simulink model "ECItoECEFtest"  (R2018a)
settings: Solver=FixedStepAuto  StartTime=0  StopTime=1*24*3600*365  FixedStep=10000  RelTol=1e-3
undefined symbols (not defined in the file or in its folder): Angle, Axis, IAU, init
libraries: robotcorelib x2, aerolibtransform2 x1, sharedtransform x1
settings Model: Creator=nathan  LastModifiedBy=nathan

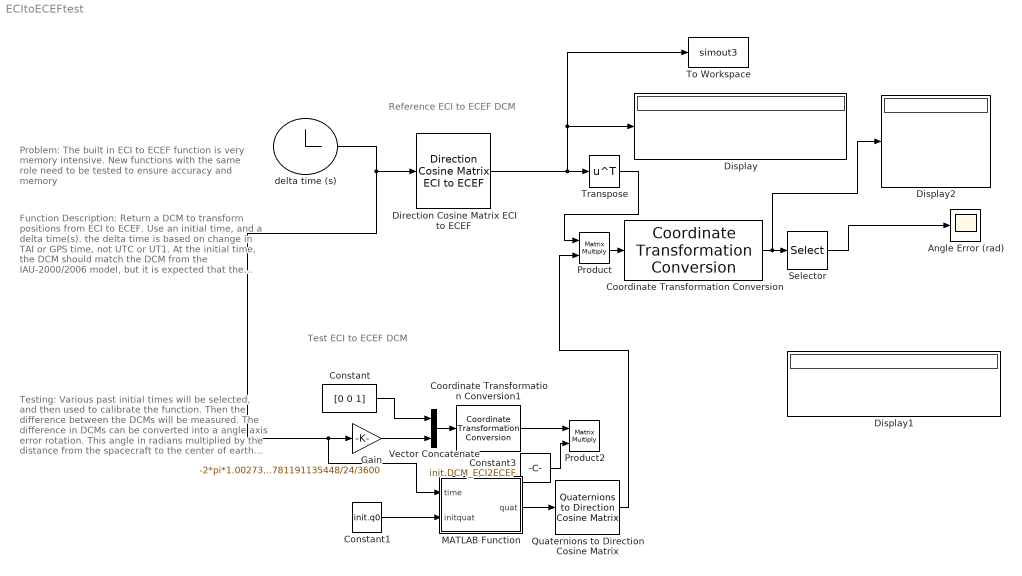
== system ECItoECEFtest ==
  note: Reference ECI to ECEF DCM
  note: Function Description:
      | Return a DCM to transform positions from ECI to ECEF. Use an initial time, and a delta time(s). the delta time is based on change in TAI or GPS time, not UTC or UT1.
      | At the initial time, the DCM should match the DCM from the IAU-2000/2006 model, but it is expected that the DCMs should slowly drift. This drift must be small enough so that in a few year from initial time, if the DCM is used to transform GPS data in ECEF to ECI, no significant error will be added.
  note: Problem:
      | The built in ECI to ECEF function is very memory intensive. New functions with the same role need to be tested to ensure accuracy and memory
  note: Testing:
      | Various past initial times will be selected, and then used to calibrate the function. Then the difference between the DCMs will be measured. The difference in DCMs can be converted into a angle axis error rotation. This angle in radians multiplied by the distance from the spacecraft to the center of earth will give the maximum offset in distance that the transform added.
  note: Test ECI to ECEF DCM
  Angle Error (rad) : Scope
  Constant : Constant  Value=[0 0 1]
  Constant1 : Constant  Value=init.q0  VectorParams1D=off
  Constant3 : Constant  Value=init.DCM_ECI2ECEF
  Coordinate Transformation Conversion : robotcorelib/Coordinate Transformation Conversion  InputRepresentation=Rotation Matrix  InputEulerSequence=ZYX  ShowTrVecInputPort=on  OutputRepresentation=Axis-Angle  OutputEulerSequence=ZYX  ShowTrVecOutputPort=on  SimulateUsing=Interpreted execution
      settings: SourceProductBaseCode=RO
  Coordinate Transformation Conversion1 : robotcorelib/Coordinate Transformation Conversion  InputRepresentation=Axis-Angle  InputEulerSequence=ZYX  ShowTrVecInputPort=on  OutputRepresentation=Rotation Matrix  OutputEulerSequence=ZYX  ShowTrVecOutputPort=on  SimulateUsing=Interpreted execution
      settings: SourceProductBaseCode=RO
  Direction Cosine Matrix ECI to ECEF : aerolibtransform2/Direction Cosine Matrix ECI to ECEF  red=IAU-2000/2006  year=2017  month=October  day=20  hour=0  min=0  sec=0  deltaT=Sec  errorflag=Error  extraparamflag=off
      settings: AttributesFormatString=%<red>  SourceProductName=Aerospace Blockset  SourceProductBaseCode=AE
  Display : Display
  Display1 : Display
  Display2 : Display
  Gain : Gain  Gain=-2*pi*1.00273781191135448/24/3600
  MATLAB Function : MATLAB Function  TreatAsAtomicUnit=on
  Product : Product  Multiplication=Matrix(*)
  Product2 : Product  Multiplication=Matrix(*)
  Quaternions to Direction Cosine Matrix : sharedtransform/Quaternions to  Direction Cosine Matrix  aMode=aMode
      settings: SourceProductName=Aerospace Blockset  SourceProductBaseCode=AE
  Selector : Selector  InputPortWidth=4  IndexOptions=Index vector (dialog)  Indices=[4]  OutputSizes=1
  To Workspace : ToWorkspace  VariableName=simout3  SaveFormat=Timeseries  SampleTime=-1
  Transpose : Math  Operator=transpose  SaturateOnIntegerOverflow=on
  Vector Concatenate : Concatenate
  delta time (s) : Clock
  wires:
  Transpose/1 -> Product/1
  Coordinate Transformation Conversion/1 -> Display2/1, Selector/1
  Product/1 -> Coordinate Transformation Conversion/1
  Selector/1 -> Angle Error (rad)/1
  Direction Cosine Matrix ECI to ECEF/1 -> To Workspace/1, Display/1, Transpose/1
  delta time (s)/1 -> MATLAB Function/1(time), Gain/1, Direction Cosine Matrix ECI to ECEF/1
  Gain/1 -> Vector Concatenate/2
  Constant1/1 -> MATLAB Function/2(initquat)
  Vector Concatenate/1 -> Coordinate Transformation Conversion1/1
  Coordinate Transformation Conversion1/1 -> Product2/1
  Constant3/1 -> Product2/2
  Constant/1 -> Vector Concatenate/1
  MATLAB Function/1(quat) -> Quaternions to Direction Cosine Matrix/1
  Quaternions to Direction Cosine Matrix/1 -> Product/2

== matlab function ECItoECEFtest/MATLAB Function ==
  data: time input; quat output; initquat input
function quat = fastquat_eci2ecef(time, initquat)
%quat_eci2ecef Returns the quaternion to rotate vectors from eci to ecef
%   time(positive float): units seconds
%   initquat(unit quaternion, 1st component real): initial quat_eci2ecef at time=0
th=2*pi*1.00273781191135448/24/3600*time;
qt= [cos(th/2) 0 0 sin(th/2)];
quat= quatmultiply(initquat,qt);
